simulink model "neuron_exc_type"  (R2022a)
settings: Solver=VariableStepAuto  StartTime=0.0  StopTime=8  RelTol=1e-3
undefined symbols (not defined in the file or in its folder): sigbuilder_block
libraries: neuromorphic_blocks x6
settings Model: Creator=chris  LastModifiedBy=chris

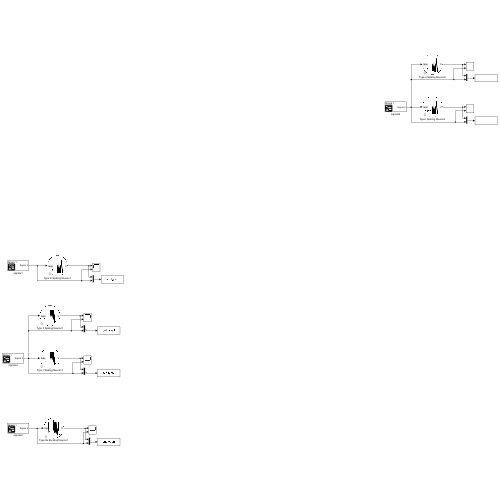
[thumbnail: Simulink's stored preview of the top-level diagram]
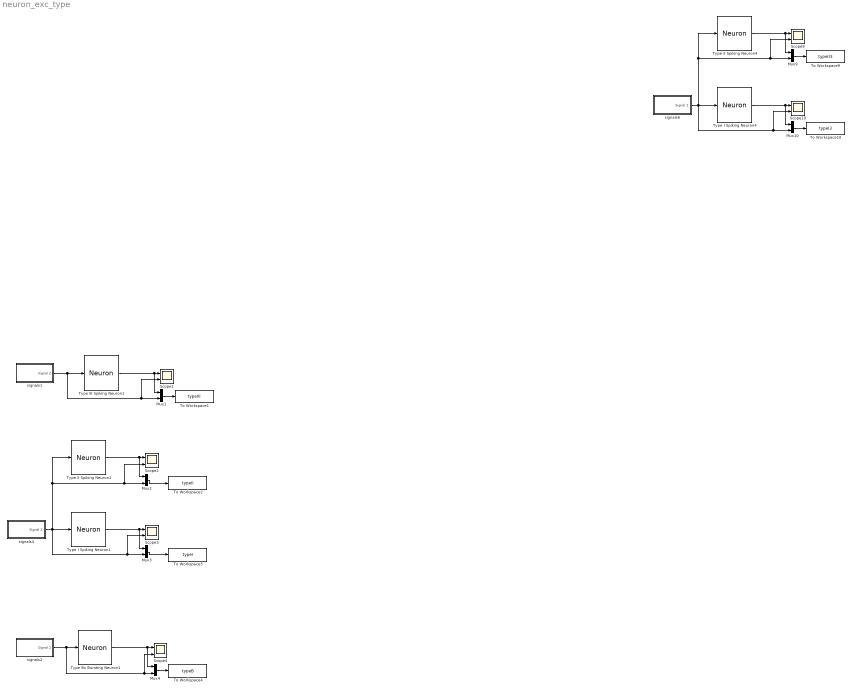
== system neuron_exc_type ==
  Mux{1..4,9..10} (6 alike) : Mux  Inputs=2
  Scope{1..4,9..10} (6 alike) : Scope  NumInputPorts=2
  To Workspace1 : ToWorkspace  VariableName=typeIII  SaveFormat=Structure With Time  SampleTime=-1
  To Workspace10 : ToWorkspace  VariableName=typeI3  SaveFormat=Structure With Time  SampleTime=-1
  To Workspace2 : ToWorkspace  VariableName=typeII  SaveFormat=Structure With Time  SampleTime=-1
  To Workspace3 : ToWorkspace  VariableName=typeI  SaveFormat=Structure With Time  SampleTime=-1
  To Workspace4 : ToWorkspace  VariableName=typeB  SaveFormat=Structure With Time  SampleTime=-1
  To Workspace9 : ToWorkspace  VariableName=typeII3  SaveFormat=Structure With Time  SampleTime=-1
  Type Bs Bursting Neuron1 : neuromorphic_blocks/Neural Blocks/Neuron  gfm_source=Internal  gfm=2  gsp_source=Internal  gsp=4  gsm_source=Internal  gsm=2  gup_source=Internal  gup=1.4  gum_source=Internal  gum=0  dfm=0  dsp=0.5  dsm=-0.5  dup=-0.5  dum=-1  mfm=1  msp=1  msm=1  mup=1  mum=1  timescale=0.004  rel_membrane=0.1  rel_fast=0.1  rel_slow=sqrt(10)  rel_ultraslow=100  Iapp_base=-0.2  V0=-1.2  tresh=0  output=Voltage
      settings: SourceProductName=Neuromorphic Toolbox
  Type I Spiking Neuron1 : neuromorphic_blocks/Neural Blocks/Neuron  gfm_source=Internal  gfm=2  gsp_source=Internal  gsp=4  gsm_source=Internal  gsm=1  gup_source=Internal  gup=0  gum_source=Internal  gum=0  dfm=0  dsp=0.5  dsm=-0.5  dup=-0.5  dum=-1  mfm=1  msp=1  msm=1  mup=1  mum=1  timescale=0.004  rel_membrane=0.1  rel_fast=0.1  rel_slow=sqrt(10)  rel_ultraslow=100  Iapp_base=-0.12  V0=-1.2  tresh=0  output=Voltage
      settings: SourceProductName=Neuromorphic Toolbox
  Type I Spiking Neuron4 : neuromorphic_blocks/Neural Blocks/Neuron  gfm_source=Internal  gfm=2  gsp_source=Internal  gsp=4  gsm_source=Internal  gsm=1  gup_source=Internal  gup=0  gum_source=Internal  gum=0  dfm=0  dsp=0.5  dsm=-0.5  dup=-0.5  dum=-1  mfm=1  msp=1  msm=1  mup=1  mum=1  timescale=0.004  rel_membrane=0.1  rel_fast=0.1  rel_slow=10  rel_ultraslow=100  Iapp_base=-0.12  V0=-1.2  tresh=0  output=Voltage
      settings: SourceProductName=Neuromorphic Toolbox
  Type II Spiking Neuron1 : neuromorphic_blocks/Neural Blocks/Neuron  gfm_source=Internal  gfm=2  gsp_source=Internal  gsp=4  gsm_source=Internal  gsm=0  gup_source=Internal  gup=0  gum_source=Internal  gum=0  dfm=0  dsp=0.5  dsm=-0.5  dup=-0.5  dum=-1  mfm=1  msp=1  msm=1  mup=1  mum=1  timescale=0.004  rel_membrane=0.1  rel_fast=0.1  rel_slow=sqrt(10)  rel_ultraslow=100  Iapp_base=0.151  V0=-1.2  tresh=0  output=Voltage
      settings: SourceProductName=Neuromorphic Toolbox
  Type II Spiking Neuron4 : neuromorphic_blocks/Neural Blocks/Neuron  gfm_source=Internal  gfm=2  gsp_source=Internal  gsp=4  gsm_source=Internal  gsm=0  gup_source=Internal  gup=0  gum_source=Internal  gum=0  dfm=0  dsp=0.5  dsm=-0.5  dup=-0.5  dum=-1  mfm=1  msp=1  msm=1  mup=1  mum=1  timescale=0.004  rel_membrane=0.1  rel_fast=0.1  rel_slow=10  rel_ultraslow=100  Iapp_base=0.132  V0=-1.2  tresh=0  output=Voltage
      settings: SourceProductName=Neuromorphic Toolbox
  Type III Spiking Neuron1 : neuromorphic_blocks/Neural Blocks/Neuron  gfm_source=Internal  gfm=2  gsp_source=Internal  gsp=4  gsm_source=Internal  gsm=0  gup_source=Internal  gup=15  gum_source=Internal  gum=0  dfm=0  dsp=0.5  dsm=-0.5  dup=-0.5  dum=-1  mfm=1  msp=1  msm=1  mup=1  mum=1  timescale=0.004  rel_membrane=0.1  rel_fast=0.1  rel_slow=sqrt(10)  rel_ultraslow=100  Iapp_base=0.1  V0=-1.2  tresh=0  output=Voltage
      settings: SourceProductName=Neuromorphic Toolbox
  signals1 : Subsystem  Tag=STV Subsys  LoadFcn=sigbuilder_block('load');  StartFcn=sigbuilder_block('start');  StopFcn=sigbuilder_block('stop');  ClipboardFcn=sigbuilder_block('clipboard');  mask(Sigbuilder block){tuvar=[0:10]}
      mask help: Simulink:masks:SigbuilderBlock_MD
      mask init:
      | if ~strcmp(get_param(bdroot(gcbh),'SimulationStatus'),'stopped') tuvar = sigbuilder_block('maskInit'); end
      settings: CopyFcn=sigbuilder_block('copy');  DeleteFcn=sigbuilder_block('delete');  ModelCloseFcn=sigbuilder_block('modelClose');  PreSaveFcn=sigbuilder_block('preSave');  PauseFcn=sigbuilder_block('pause');  ContinueFcn=sigbuilder_block('continue');  NameChangeFcn=sigbuilder_block('namechange');  OpenFcn=sigbuilder_block('open',[822.75 417 550.5 364.5 ]);  CloseFcn=sigbuilder_block('close');
      mask Display: plot(0, 0, 100, 100,[2, 2, 32, 32, 2], [68, 8, 8, 68, 68],[32, 2], [38, 38], [32, 19, 2],[53, 60, 44], [32, 17, 17, 2],[16, 16, 31, 31]);txt = getActiveGroup(gcbh);text(2, 100, txt,'verticalAlignment', 'top');
  signals2 : Subsystem  Tag=STV Subsys  LoadFcn=sigbuilder_block('load');  StartFcn=sigbuilder_block('start');  StopFcn=sigbuilder_block('stop');  ClipboardFcn=sigbuilder_block('clipboard');  mask(Sigbuilder block){tuvar=[0:10]}
      mask help: Simulink:masks:SigbuilderBlock_MD
      mask init:
      | if ~strcmp(get_param(bdroot(gcbh),'SimulationStatus'),'stopped') tuvar = sigbuilder_block('maskInit'); end
      settings: CopyFcn=sigbuilder_block('copy');  DeleteFcn=sigbuilder_block('delete');  ModelCloseFcn=sigbuilder_block('modelClose');  PreSaveFcn=sigbuilder_block('preSave');  PauseFcn=sigbuilder_block('pause');  ContinueFcn=sigbuilder_block('continue');  NameChangeFcn=sigbuilder_block('namechange');  OpenFcn=sigbuilder_block('open',[716.625 468.75 718.5 338.25 ]);  CloseFcn=sigbuilder_block('close');
      mask Display: plot(0, 0, 100, 100,[2, 2, 32, 32, 2], [68, 8, 8, 68, 68],[32, 2], [38, 38], [32, 19, 2],[53, 60, 44], [32, 17, 17, 2],[16, 16, 31, 31]);txt = getActiveGroup(gcbh);text(2, 100, txt,'verticalAlignment', 'top');
  signals4 : Subsystem  Tag=STV Subsys  LoadFcn=sigbuilder_block('load');  StartFcn=sigbuilder_block('start');  StopFcn=sigbuilder_block('stop');  ClipboardFcn=sigbuilder_block('clipboard');  mask(Sigbuilder block){tuvar=[0:10]}
      mask help: Simulink:masks:SigbuilderBlock_MD
      mask init:
      | if ~strcmp(get_param(bdroot(gcbh),'SimulationStatus'),'stopped') tuvar = sigbuilder_block('maskInit'); end
      settings: CopyFcn=sigbuilder_block('copy');  DeleteFcn=sigbuilder_block('delete');  ModelCloseFcn=sigbuilder_block('modelClose');  PreSaveFcn=sigbuilder_block('preSave');  PauseFcn=sigbuilder_block('pause');  ContinueFcn=sigbuilder_block('continue');  NameChangeFcn=sigbuilder_block('namechange');  OpenFcn=sigbuilder_block('open',[239.625 94.5 550.5 364.5 ]);  CloseFcn=sigbuilder_block('close');
      mask Display: plot(0, 0, 100, 100,[2, 2, 32, 32, 2], [68, 8, 8, 68, 68],[32, 2], [38, 38], [32, 19, 2],[53, 60, 44], [32, 17, 17, 2],[16, 16, 31, 31]);txt = getActiveGroup(gcbh);text(2, 100, txt,'verticalAlignment', 'top');
  signals6 : Subsystem  Tag=STV Subsys  LoadFcn=sigbuilder_block('load');  StartFcn=sigbuilder_block('start');  StopFcn=sigbuilder_block('stop');  ClipboardFcn=sigbuilder_block('clipboard');  mask(Sigbuilder block){tuvar=[0:10]}
      mask help: Simulink:masks:SigbuilderBlock_MD
      mask init:
      | if ~strcmp(get_param(bdroot(gcbh),'SimulationStatus'),'stopped') tuvar = sigbuilder_block('maskInit'); end
      settings: CopyFcn=sigbuilder_block('copy');  DeleteFcn=sigbuilder_block('delete');  ModelCloseFcn=sigbuilder_block('modelClose');  PreSaveFcn=sigbuilder_block('preSave');  PauseFcn=sigbuilder_block('pause');  ContinueFcn=sigbuilder_block('continue');  NameChangeFcn=sigbuilder_block('namechange');  OpenFcn=sigbuilder_block('open',[239.625 94.5 550.5 364.5 ]);  CloseFcn=sigbuilder_block('close');
      mask Display: plot(0, 0, 100, 100,[2, 2, 32, 32, 2], [68, 8, 8, 68, 68],[32, 2], [38, 38], [32, 19, 2],[53, 60, 44], [32, 17, 17, 2],[16, 16, 31, 31]);txt = getActiveGroup(gcbh);text(2, 100, txt,'verticalAlignment', 'top');
  wires:
  signals1/1(Signal 2) -> Type III Spiking Neuron1/1, Mux1/2, Scope1/2
  Type III Spiking Neuron1/1 -> Mux1/1, Scope1/1
  Mux1/1 -> To Workspace1/1
  signals2/1(Signal 2) -> Type Bs Bursting Neuron1/1, Scope4/2, Mux4/2
  Type Bs Bursting Neuron1/1 -> Mux4/1, Scope4/1
  Mux4/1 -> To Workspace4/1
  Type I Spiking Neuron4/1 -> Mux10/1, Scope10/1
  Mux9/1 -> To Workspace9/1
  Mux10/1 -> To Workspace10/1
  Type II Spiking Neuron4/1 -> Mux9/1, Scope9/1
  signals6/1(Signal 2) -> Type II Spiking Neuron4/1, Scope9/2, Mux9/2, Mux10/2, Scope10/2, Type I Spiking Neuron4/1
  signals4/1(Signal 2) -> Type II Spiking Neuron1/1, Scope2/2, Mux2/2, Mux3/2, Scope3/2, Type I Spiking Neuron1/1
  Type II Spiking Neuron1/1 -> Mux2/1, Scope2/1
  Type I Spiking Neuron1/1 -> Mux3/1, Scope3/1
  Mux3/1 -> To Workspace3/1
  Mux2/1 -> To Workspace2/1

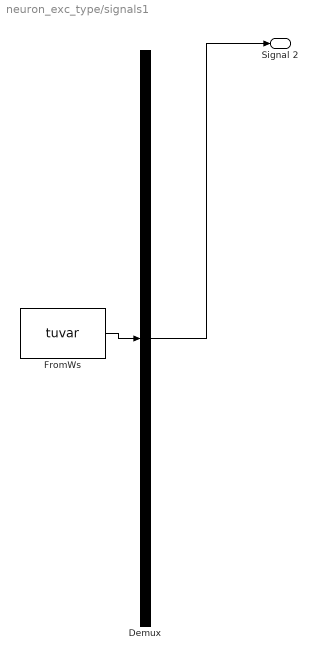
== system neuron_exc_type/signals1 ==
  Demux : Demux  Tag=STV Demux  Outputs=1
      settings: DisplayOption=none
  FromWs : FromWorkspace  Tag=STV FromWs  VariableName=tuvar  OutputAfterFinalValue=Holding final value
      SigBuilderData=|
      | common.afterFinalStr = 'Hold final value'
      | common.sampleTime = '0'
      | dataSet.timeRange = [0 10]
      | dataSet.name = 'Group 1'
      | sbobj.Groups.Name = 'Group 1'
      | sbobj.Groups.Signals.Name = 'Signal 2'
      | sbobj.Groups.Signals.XData = [0 2 2 2.5 2.5 2.9 2.9 3 3 10]
      | sbobj.Groups.Signals.YData = [0 0 0.2 0.2 0 0 -0.3 -0.3 0 0]
  Signal 2 : Outport  Tag=STV Outport
  wires:
  FromWs/1 -> Demux/1
  Demux/1 -> Signal 2/1

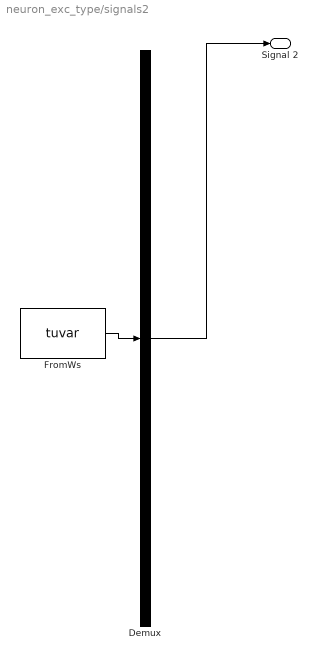
== system neuron_exc_type/signals2 ==
  Demux : Demux  Tag=STV Demux  Outputs=1
      settings: DisplayOption=none
  FromWs : FromWorkspace  Tag=STV FromWs  VariableName=tuvar  OutputAfterFinalValue=Holding final value
      SigBuilderData=|
      | common.afterFinalStr = 'Hold final value'
      | common.sampleTime = '0'
      | dataSet.timeRange = [0 10]
      | dataSet.name = 'Group 1'
      | sbobj.Groups.Name = 'Group 1'
      | sbobj.Groups.Signals.Name = 'Signal 2'
      | sbobj.Groups.Signals.XData = [0 2 2 2.9 2.9 3.4 3.4 3.45 3.45 3.9 3.9 4 4 10]
      | sbobj.Groups.Signals.YData = [0 0 0.2 0.2 0 0 0.2 0.2 0 0 -0.4 -0.4 0 0]
  Signal 2 : Outport  Tag=STV Outport
  wires:
  FromWs/1 -> Demux/1
  Demux/1 -> Signal 2/1

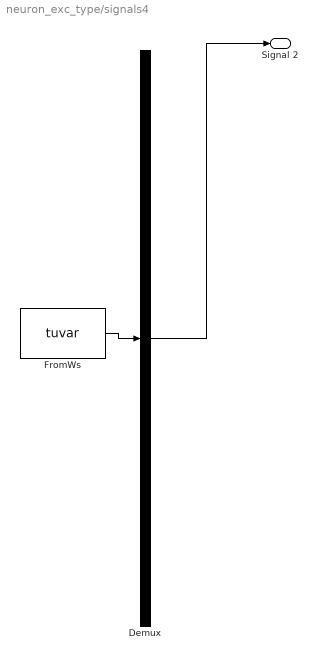
== system neuron_exc_type/signals4 ==
  Demux : Demux  Tag=STV Demux  Outputs=1
      settings: DisplayOption=none
  FromWs : FromWorkspace  Tag=STV FromWs  VariableName=tuvar  OutputAfterFinalValue=Holding final value
      SigBuilderData=|
      | common.afterFinalStr = 'Hold final value'
      | common.sampleTime = '0'
      | dataSet.timeRange = [0 10]
      | dataSet.name = 'Group 1'
      | sbobj.Groups.Name = 'Group 1'
      | sbobj.Groups.Signals.Name = 'Signal 2'
      | sbobj.Groups.Signals.XData = [0 2 2 2.5 2.5 3 3 3.5 3.5 4 4 4.0125 4.0125 4.5 4.5 4.6 4.6 10]
      | sbobj.Groups.Signals.YData = [0 0 0.163 0.163 0 0 0.18 0.18 0 0 0.2 0.2 0 0 -0.3 -0.3 0 0]
  Signal 2 : Outport  Tag=STV Outport
  wires:
  FromWs/1 -> Demux/1
  Demux/1 -> Signal 2/1

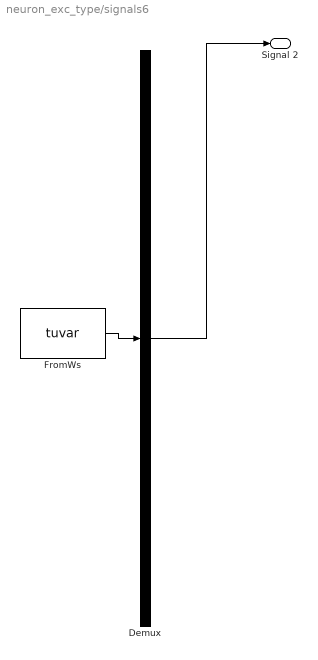
== system neuron_exc_type/signals6 ==
  Demux : Demux  Tag=STV Demux  Outputs=1
      settings: DisplayOption=none
  FromWs : FromWorkspace  Tag=STV FromWs  VariableName=tuvar  OutputAfterFinalValue=Holding final value
      SigBuilderData=|
      | common.afterFinalStr = 'Hold final value'
      | common.sampleTime = '0'
      | dataSet.timeRange = [0 10]
      | dataSet.name = 'Group 1'
      | sbobj.Groups.Name = 'Group 1'
      | sbobj.Groups.Signals.Name = 'Signal 2'
      | sbobj.Groups.Signals.XData = [0 2 2 4.7 4.7 5 5 5.025 5.025 5.5 5.5 5.525 5.525 10]
      | sbobj.Groups.Signals.YData = [0 0 0.162 0.167 0 0 0.2 0.2 0 0 -0.6 -0.6 0 0]
  Signal 2 : Outport  Tag=STV Outport
  wires:
  FromWs/1 -> Demux/1
  Demux/1 -> Signal 2/1
